simulink model "Simulator"  (R2024a)
settings: Solver=VariableStepAuto  StartTime=0.0  StopTime=inf  RelTol=1e-5
values from neighbouring files (symbols this model uses):
  I = [3000 0 0 ... (first row only)    [Constants_gui.m]    (also in constants.m; mbi.m = [15, .25, .20; set_up_HW7.m = I-Id; setupConstantRateSDA.m)
  invI = inv(I)    [Constants_gui.m]    (also in constants.m; mbi.m; set_up_HW7.m; setupConstantRateSDA.m)
  q_init = q_init/norm(q_init)    [Constants_gui.m]    (also in constants.m = [-0.5 -0.5 -0.5 0.5]; mbi.m = [0 0 0 1]'; set_up_HW7.m = [0 0 0 1]'; setupConstantRateSDA.m)
  wbn_init = pi/30*[0 0 0]'    [Constants_gui.m]    (also in constants.m = pi/180 * [0.1; 0.2; 0.15]; mbi.m = [0 0 0]'; set_up_HW7.m = pi/30*[0 0 .01]'; setupConstantRateSDA.m)
  wn = 0.01    [Constants_gui.m]    (also in constants.m = 0.05; setupConstantRateSDA.m = 0.05)
  zet = .7071    (= 0.7071)    [Constants_gui.m]    (also in constants.m; setupConstantRateSDA.m)
undefined symbols (not defined in the file or in its folder): w_init
libraries: sharedtransform x6, aerolibutil x5, sharedutil x2, simulink x2, dspinverses x1
(part 1 of 4)
settings Model: Creator=nidhisonwalkar  LastModifiedBy=robertbergbaum

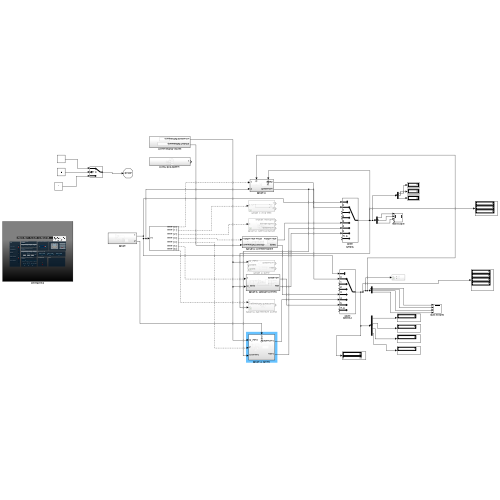
[thumbnail: Simulink's stored preview of the top-level diagram]
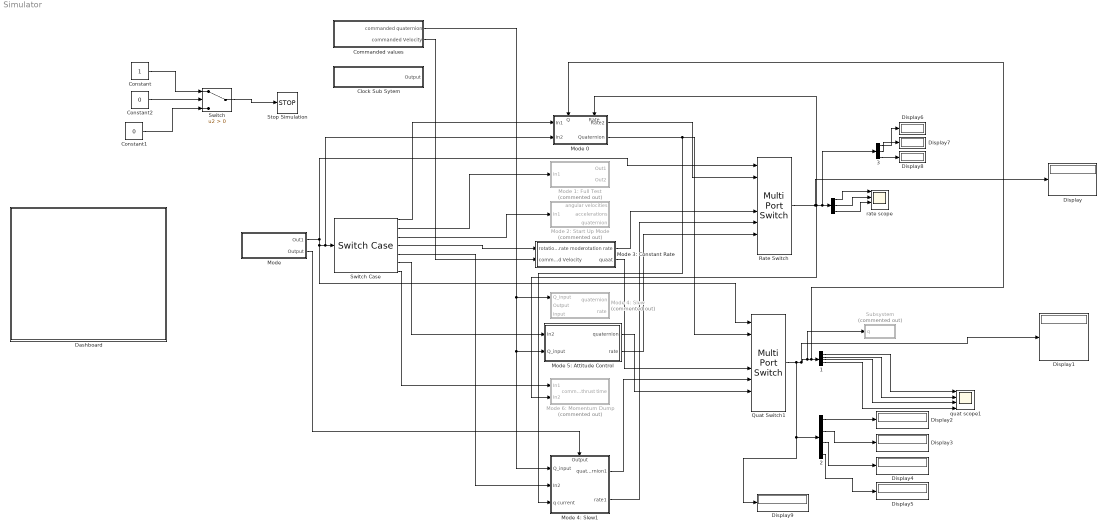
== system Simulator ==
  " " : Demux  Outputs=3
      settings: DisplayOption=none
  " 1" : Demux
      settings: DisplayOption=none
  " 2" : Demux
      settings: DisplayOption=none
  " 3" : Demux  Outputs=3
      settings: DisplayOption=none
  "Clock Sub Sytem " : Subsystem
  Commanded values : Subsystem
  Constant : Constant
  Constant1 : Constant  Value=0
  Constant2 : Constant  Value=0
  Dashboard : Subsystem
  Display{,1..9} (10 alike) : Display
  Mode : Subsystem
  "Mode 0 " : Subsystem
      settings: PortSchema="{\"entries\":[{\"content\":{\"sides\":[{\"content\":{\"connectorIds\":[\"In1\",\"In2\"]},\"type\":\"ConnectorPlacement.EquallySpacedRectSide\",\"uuid\":\"86d363f2-53dc-4b23-b557-4d4fa5837e38\"},{\"content\":{\"connectorIds\":[\"Out1\",\"Out2\"],\"side\":\"RIGHT\"},\"type\":\"ConnectorPlacement.EquallySpacedRectSide\",\"uuid\":\"eedbdfbc-6d02-4f31-9c03-399fb804b597\"},{\"content\":{\"connectorIds\":[\"In3\",\"In4\"],\"side\":\"TOP\"},\"type\":\"ConnectorPlacement.EquallySpacedRectSide\",\"uuid\":\"84da8539-1f14-466f-849c-27e820ab14ca\"}]},\"type\":\"ConnectorPlacement.EquallySpacedConnector\",\"uuid\":\"554c5755-9926-49c6-9537-0be488121aec\"}],\"packageUris\":[\"http://schema.mathworks.com/mf0/Connector/R2020b\"],\"version\":\"1.0\"}"
  Mode 1: Full Test : Subsystem  Commented=on
  Mode 2: Start Up Mode : Subsystem  Commented=on
  Mode 3: Constant Rate : Subsystem
  Mode 4: Slew : Subsystem  Commented=on
  Mode 4: Slew1 : Subsystem
      settings: PortSchema="{\"entries\":[{\"content\":{\"sides\":[{\"content\":{\"connectorIds\":[\"In1\",\"In2\",\"In3\"]},\"type\":\"ConnectorPlacement.EquallySpacedRectSide\",\"uuid\":\"5aa46160-cab8-4455-8c50-72002a12dc6a\"},{\"content\":{\"connectorIds\":[\"Out1\",\"Out2\"],\"side\":\"RIGHT\"},\"type\":\"ConnectorPlacement.EquallySpacedRectSide\",\"uuid\":\"d2369968-ae02-4f92-82b5-f3bde6d13a0e\"},{\"content\":{\"connectorIds\":[\"In4\"],\"side\":\"TOP\"},\"type\":\"ConnectorPlacement.EquallySpacedRectSide\",\"uuid\":\"830a25ab-284f-47cd-8cef-c0c34f43eaff\"}]},\"type\":\"ConnectorPlacement.EquallySpacedConnector\",\"uuid\":\"052ced75-77db-4eba-9e99-628f75a27de2\"}],\"packageUris\":[\"http://schema.mathworks.com/mf0/Connector/R2020b\"],\"version\":\"1.0\"}"
  Mode 5: Attitude Control : Subsystem
  Mode 6: Momentum Dump : Subsystem  Commented=on
  Quat Switch1 : MultiPortSwitch  DataPortOrder=Specify indices  Inputs=6  DataPortIndices={0,1,2,3,4,5,6}  SaturateOnIntegerOverflow=off  InputSameDT=off
  Rate Switch : MultiPortSwitch  DataPortOrder=Specify indices  Inputs=6  DataPortIndices={0,1,2,3,4,5,6}  SaturateOnIntegerOverflow=off  InputSameDT=off
  Stop Simulation : Stop
  Subsystem : Subsystem  Commented=on
  Switch : Switch  Criteria=u2 > Threshold  SaturateOnIntegerOverflow=off  InputSameDT=off
  Switch Case : SwitchCase  CaseConditions={0,1, 2, 3, 4, 5, 6}  ShowDefaultCase=off
  quat scope1 : Scope  NumInputPorts=4
  rate scope : Scope  NumInputPorts=4
  wires:
  " "/1 -> rate scope/1
  " "/2 -> rate scope/2
  " "/3 -> rate scope/3
  Rate Switch/1 -> Display/1, Mode 6: Momentum Dump/2(In2), " 3"/1, " "/1, "Mode 0 "/4(Rate)
  " 1"/3 -> quat scope1/3
  " 1"/2 -> quat scope1/2
  " 1"/4 -> quat scope1/4
  " 1"/1 -> quat scope1/1
  Mode/1(Out1) -> Quat Switch1/1, "Mode 0 "/2(In2), Switch Case/1, Rate Switch/1
  Switch Case/1 -> "Mode 0 "/1(In1)
  Switch Case/2 -> Mode 1: Full Test/1(In1)
  Switch Case/3 -> Mode 2: Start Up Mode/1(In1)
  Switch Case/4 -> Mode 3: Constant Rate/1(rotation rate mode)
  Switch Case/7 -> Mode 6: Momentum Dump/1(In1)
  "Mode 0 "/1(Rate2) -> Rate Switch/2
  Commanded values/2(commanded Velocity) -> Mode 3: Constant Rate/2(commanded Velocity)
  Mode 3: Constant Rate/1(rotation rate) -> Rate Switch/5
  Mode 3: Constant Rate/2("quaat ") -> Quat Switch1/5
  Commanded values/1(commanded quaternion) -> Mode 4: Slew1/1(Q_input), Mode 5: Attitude Control/2(Q_input), Mode 4: Slew/1(Q_input)
  Switch Case/6 -> Mode 5: Attitude Control/1(In2)
  Mode 5: Attitude Control/2(rate) -> Rate Switch/7
  Mode 5: Attitude Control/1(quaternion) -> Quat Switch1/7
  " 2"/4 -> Display5/1
  " 2"/1 -> Display2/1
  " 2"/2 -> Display3/1
  " 2"/3 -> Display4/1
  " 3"/1 -> Display6/1
  " 3"/2 -> Display7/1
  " 3"/3 -> Display8/1
  Switch/1 -> Stop Simulation/1
  Constant/1 -> Switch/1
  Constant1/1 -> Switch/3
  Constant2/1 -> Switch/2
  Mode/2(Output) -> Mode 4: Slew1/4(Output)
  Mode 4: Slew1/2(rate1) -> Rate Switch/6
  Quat Switch1/1 -> Display9/1, " 2"/1, Display1/1, "Mode 0 "/3(Q), " 1"/1, Subsystem/1(q)
  Mode 4: Slew1/1(quaternion1) -> Quat Switch1/6
  "Mode 0 "/2(Quaternion) -> Mode 4: Slew1/3(q current), Quat Switch1/2
  Switch Case/5 -> Mode 4: Slew1/2(In2)

== system Simulator/Clock Sub Sytem  ==
  Clock : Clock
  Clock1 : Clock
  Clock2 : Clock
  Display : Display
  Display1 : Display
  Display2 : Display
  Gain : Gain
  Gain1 : Gain  Gain=3600
  Output : Outport
  wires:
  Gain1/1 -> Display2/1
  Clock/1 -> Output/1, Display/1
  Clock2/1 -> Gain/1
  Clock1/1 -> Gain1/1
  Gain/1 -> Display1/1

== system Simulator/Commanded values ==
  Commanded Quaternion : Subsystem
  Commanded Velocity : Subsystem
  commanded quaternion : Outport
  commanded Velocity : Outport  Port=2
  wires:
  Commanded Velocity/1(Out1) -> commanded Velocity/1
  Commanded Quaternion/1(Out1) -> commanded quaternion/1
